simulink model "fun"  (R2023b)
settings: Solver=FixedStepAuto  StartTime=0.0  StopTime=10  FixedStep=1  RelTol=1e-3
settings Model: FPTShortcutValueString='{{},{''BaselineRun_3'',1,1,1,''BaselineRun_3'','''',{},''M'',''D'',''''},{''EmbeddedRun'',1,1,1,''EmbeddedRun'','''',{},''M'','''',''''},{''EmbeddedRun_2'',1,1,1,''EmbeddedRun_2'','''',{},''M'','''',''''},{''EmbeddedRun_3'',1,1,1,''EmbeddedRun_3'','''',{},''M'','''',''''}}'  Creator=qasem  LastModifiedBy=Fartash
settings OptimizationCC: DefaultParameterBehavior=Inlined  EnhancedBackFolding=on  PassReuseOutputArgsAs=Individual arguments  InitFltsAndDblsToZero=on  OptimizeBlockOrder=speed  DifferentSizesBufferReuse=on  OptimizationCustomize=off  EfficientTunableParamExpr=on
settings DebuggingCC: SignalRangeChecking=warning  ParameterTunabilityLossMsg=error
settings HardwareCC: ProdLongLongMode=on  TargetLongLongMode=on
settings SFSimCC: MATLABDynamicMemAlloc=off
settings RTWCC: Description=Embedded Coder  SystemTargetFile=ert.tlc  GenCodeOnly=on  TemplateMakefile=ert_default_tmf  Toolchain=MinGW64 | CMake/gmake (64-bit Windows)  BuildConfiguration=Release  TargetLang=C++
settings CodeAppCC: ForceParamTrailComments=on  IgnoreCustomStorageClasses=off  OperatorAnnotations=on  SimulinkDataObjDesc=on  SFDataObjDesc=on  InsertBlockDesc=on
settings ERTTargetCC: TargetLangStandard=C++11 (ISO)  GenerateSampleERTMain=on  CodeInterfacePackaging=Reusable function  InlinedParameterPlacement=NonHierarchical  ERTCustomFileTemplate=example_file_process.tlc

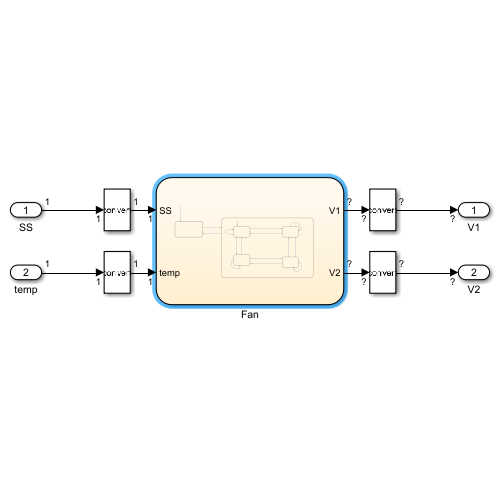
[thumbnail: Simulink's stored preview of the top-level diagram]
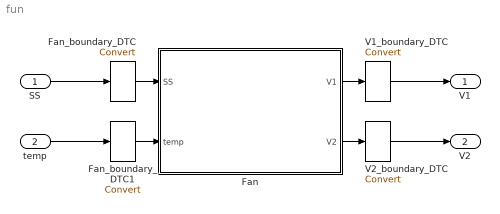
== system fun ==
  SS : Inport  OutDataTypeStr=fixdt(1,16,4)
  temp : Inport  Port=2  OutDataTypeStr=fixdt(1,16,4)
  Fan : Stateflow chart  TreatAsAtomicUnit=on
  Fan_boundary_DTC : DataTypeConversion
  Fan_boundary_DTC1 : DataTypeConversion
  V1_boundary_DTC : DataTypeConversion
  V2_boundary_DTC : DataTypeConversion
  V1 : Outport
  V2 : Outport  Port=2
  wires:
  SS/1 -> Fan_boundary_DTC/1
  Fan_boundary_DTC/1 -> Fan/1(SS)
  temp/1 -> Fan_boundary_DTC1/1
  Fan_boundary_DTC1/1 -> Fan/2(temp)
  Fan/1(V1) -> V1_boundary_DTC/1
  V1_boundary_DTC/1 -> V1/1
  Fan/2(V2) -> V2_boundary_DTC/1
  V2_boundary_DTC/1 -> V2/1

== stateflow chart fun/Fan ==
  state On
    state RightLow
      entry:
      V1  = temp - 20;
      V2 = 10;
    state RighHigh
      entry:
      V1  = temp - 20;
      V2 = 20;
    state LeftLow
      entry:
      V1  = temp - 20;
      V2 = -10;
    state LeftHigh
      entry:
      V1  = temp - 20;
      V2 = -20;
    (default) -> RightLow
    RighHigh -> RighHigh [order 3] : {counter = counter + 1;}
    RightLow -> RighHigh [order 1] : [SS == 1]
    RightLow -> RightLow [order 3] : {counter = counter +1}
    RighHigh -> RightLow [order 1] : [SS == 0]
    RightLow -> LeftLow [order 2] : [counter >= 10]{counter = 0}
    LeftLow -> RightLow [order 2] : [counter >= 10]{counter = 0}
    LeftHigh -> RighHigh [order 1] : [counter >= 5]{counter = 0}
    RighHigh -> LeftHigh [order 2] : [counter >= 5]{counter = 0}
    LeftLow -> LeftHigh [order 1] : [SS == 1]
    LeftLow -> LeftLow [order 3] : {counter = counter + 1}
    LeftHigh -> LeftHigh [order 3] : {counter = counter +1}
    LeftHigh -> LeftLow [order 2] : [SS == 0]
  state Off
    entry:
    V1 = 0;
    V2 = 0;
    counter = 0;
  (default) -> Off
  Off -> On : [temp > 20]
  On -> Off : [temp <= 20]
  data: V1 output fixdt(1,16,0); V2 output fixdt(1,16,0); SS input fixdt(1,16,0); counter local fixdt(1,16,0); temp input fixdt(1,16,0)
